simulink subsystem "DesalHydraulicsERU"  (R2025b)
settings: Solver=VariableStepAuto  StartTime=0.0  StopTime=10.0  RelTol=1e-3
libraries: customization_lib x22, nesl_utility x10, fl_lib x1
settings Model: Creator=ndegoede  LastModifiedBy=degoede

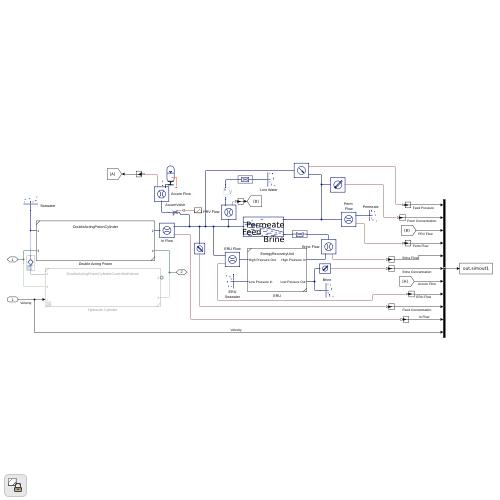
[thumbnail: Simulink's stored preview of the top-level diagram]
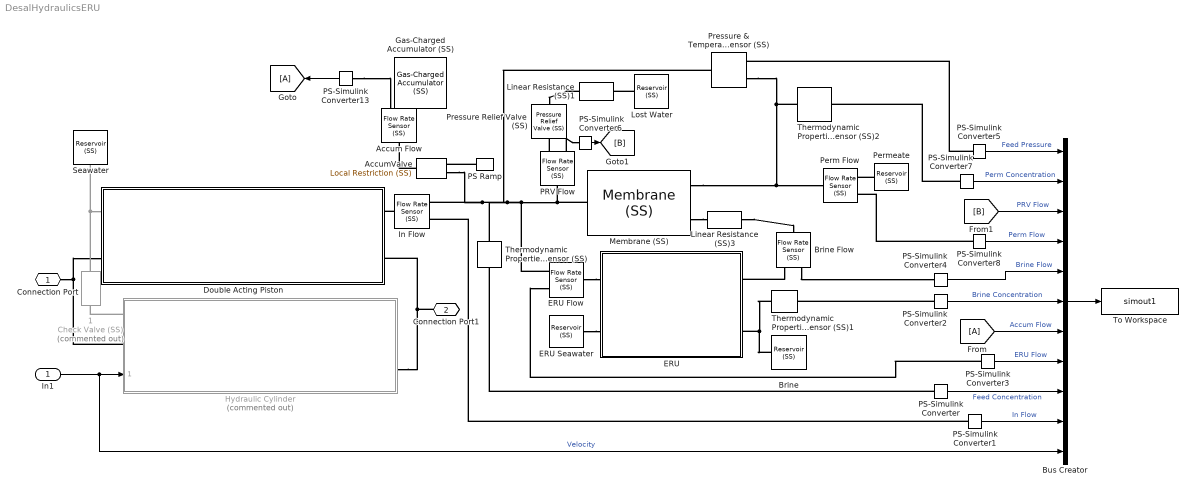
== system DesalHydraulicsERU ==
  In1 : Inport
  " Seawater" : customization_lib/solution/elements/Reservoir (SS)  pressure_spec=foundation.enum.pressure_spec.specified  reservoir_pressure=0.2 MPa  reservoir_temperature=293.15 K  reservoir_concentration=36 kg/m^3  reservoir_concentration_y=0 kg/m^3  reservoir_concentration_z=0 kg/m^3  area=0.01 m^2  custom_ports=false  length_A=1e-3 m
      settings: SourceProductName=Customization  InternalSimscapePortConfiguration="{\"Bottom\":[],\"Left\":[{\"id\":\"A\",\"label\":\"A\",\"type\":\"customization.solution.solution\"}],\"Right\":[],\"Top\":[]}"
  " 1" : customization_lib/solution/elements/Check Valve (SS)  Commented=on  opening_spec=fluids.thermal_liquid.valves.enum.PressureOpeningSpec.Linear  pressure_spec=fluids.thermal_liquid.valves.enum.PressureControlSpec.PressureDifferential  p_crack_gauge=0.1 MPa  p_crack_differential=0.01 MPa  press_max_gauge=0.2 MPa  press_max_differential=0.02 MPa  area_max=0.05 m^2  area_leak=1e-8 m^2  p_diff_TLU=[0.01 : 0.01 : 0.1] MPa  valve_area_TLU=[1e-10, 1e-05, 2e-05, 3e-05, 4e-05, 5e-05, 6e-05, 7.5e-05, 8.5e-05, .0001] m^2  vol_flow_TLU=[.000358, .045, .11, .191, .284, .39, .505, .63, .764, .905] .* 1e-3 m^3/s  area=0.1 m^2  Cd=0.7  Re_c=150  smoothing_factor=0.01  pressure_recovery=false  opening_dynamics=false  tau=0.1 s  custom_ports=false  length_A=1e-3 m  length_B=1e-3 m
      settings: SourceProductName=Customization  InternalSimscapePortConfiguration="{\"Bottom\":[],\"Left\":[{\"id\":\"A\",\"label\":\"A\",\"type\":\"customization.solution.solution\"}],\"Right\":[{\"id\":\"B\",\"label\":\"B\",\"type\":\"customization.solution.solution\"}],\"Top\":[]}"
  Accum Flow : customization_lib/solution/sensors/Flow Rate Sensor (SS)  mass_flow_measure=false  volumetric_flow_measure=true  solute_flow_measure=false  solute_y_flow_measure=false  solute_z_flow_measure=false  energy_flow_measure=false
      settings: SourceProductName=Customization  InternalSimscapePortConfiguration="{\"Bottom\":[],\"Left\":[{\"id\":\"A\",\"label\":\"A\",\"type\":\"customization.solution.solution\"}],\"Right\":[{\"id\":\"B\",\"label\":\"B\",\"type\":\"customization.solution.solution\"},{\"id\":\"V\",\"label\":\"V\",\"type\":\"output\"}],\"Top\":[]}"
  AccumValve : customization_lib/solution/elements/Local Restriction (SS)  restriction_type=foundation.enum.restriction_type.variable  restriction_area=0.001 m^2  min_area=1e-8 m^2  max_area=0.05 m^2  area=0.1 m^2  Cd=0.7  Re_c=150  pressure_recovery=simscape.enum.onoff.off  custom_ports=false  length_A=1e-3 m  length_B=1e-3 m
      settings: SourceProductName=Customization  InternalSimscapePortConfiguration="{\"Bottom\":[],\"Left\":[{\"id\":\"A\",\"label\":\"A\",\"type\":\"customization.solution.solution\"},{\"id\":\"area_in\",\"label\":\"AR\",\"type\":\"input\"}],\"Right\":[{\"id\":\"B\",\"label\":\"B\",\"type\":\"customization.solution.solution\"}],\"Top\":[]}"
  Brine : customization_lib/solution/elements/Reservoir (SS)  pressure_spec=foundation.enum.pressure_spec.atmospheric  reservoir_pressure=0.101325 MPa  reservoir_temperature=293.15 K  reservoir_concentration=36 kg/m^3  reservoir_concentration_y=0 kg/m^3  reservoir_concentration_z=0 kg/m^3  area=0.1 m^2  custom_ports=true  length_A=1 m
      settings: SourceProductName=Customization  InternalSimscapePortConfiguration="{\"Bottom\":[],\"Left\":[{\"id\":\"A\",\"label\":\"A\",\"type\":\"customization.solution.solution\"}],\"Right\":[],\"Top\":[]}"
  Brine Flow : customization_lib/solution/sensors/Flow Rate Sensor (SS)  mass_flow_measure=false  volumetric_flow_measure=true  solute_flow_measure=false  solute_y_flow_measure=false  solute_z_flow_measure=false  energy_flow_measure=false
      settings: SourceProductName=Customization  InternalSimscapePortConfiguration="{\"Bottom\":[],\"Left\":[{\"id\":\"A\",\"label\":\"A\",\"type\":\"customization.solution.solution\"}],\"Right\":[{\"id\":\"B\",\"label\":\"B\",\"type\":\"customization.solution.solution\"},{\"id\":\"V\",\"label\":\"V\",\"type\":\"output\"}],\"Top\":[]}"
  Bus Creator : BusCreator  Inputs=11
  Double Acting Piston : Subsystem  ReferencedSubsystem=DoubleActingPistonCylinder
      settings: PortSchema="{\"entries\":[{\"content\":{\"sides\":[{\"content\":{\"connectorIds\":[\"LConn1\",\"LConn3\"]},\"type\":\"ConnectorPlacement.EquallySpacedRectSide\",\"uuid\":\"8acd0945-963f-4ac9-9e22-6ebef24fa469\"},{\"content\":{\"connectorIds\":[\"LConn2\",\"LConn4\"],\"side\":\"RIGHT\"},\"type\":\"ConnectorPlacement.EquallySpacedRectSide\",\"uuid\":\"3b4a74cd-deb1-4dcf-bacc-c9108daeb4d0\"},{\"content\":{\"side\":\"TOP\"},\"type\":\"ConnectorPlacement.EquallySpacedRectSide\",\"uuid\":\"b26b8698-1eb6-4b70-b966-bc7275cbd4a0\"},{\"content\":{\"side\":\"BOTTOM\"},\"type\":\"ConnectorPlacement.EquallySpacedRectSide\",\"uuid\":\"df97d8fb-7bd4-42c8-81cb-d93f7329400b\"}]},\"type\":\"ConnectorPlacement.EquallySpacedConnector\",\"uuid\":\"8ea66071-78df-4809-a2e0-9adf4b1871fd\"}],\"packageUris\":[\"http://schema.mathworks.com/mf0/Connector/R2020b\"],\"version\":\"1.0\"}"
  ERU : Subsystem  ReferencedSubsystem=EnergyRecoveryUnit
      settings: PortSchema="{\"entries\":[{\"content\":{\"sides\":[{\"content\":{\"connectorIds\":[\"LConn4\",\"LConn3\"]},\"type\":\"ConnectorPlacement.EquallySpacedRectSide\",\"uuid\":\"dfa76b21-2359-4361-afcd-412f59dbf2f7\"},{\"content\":{\"connectorIds\":[\"LConn1\",\"LConn2\"],\"side\":\"RIGHT\"},\"type\":\"ConnectorPlacement.EquallySpacedRectSide\",\"uuid\":\"8a873e0a-23e4-4021-8054-e473ffd3fddb\"},{\"content\":{\"side\":\"TOP\"},\"type\":\"ConnectorPlacement.EquallySpacedRectSide\",\"uuid\":\"dbbe8b32-d4e5-4ced-b70e-6884432bc55a\"}]},\"type\":\"ConnectorPlacement.EquallySpacedConnector\",\"uuid\":\"6b5e7d52-c55b-4be9-b32d-a2c1e9796720\"}],\"packageUris\":[\"http://schema.mathworks.com/mf0/Connector/R2020b\"],\"version\":\"1.0\"}"
  ERU Seawater : customization_lib/solution/elements/Reservoir (SS)  pressure_spec=foundation.enum.pressure_spec.atmospheric  reservoir_pressure=1 MPa  reservoir_temperature=293.15 K  reservoir_concentration=36 kg/m^3  reservoir_concentration_y=0 kg/m^3  reservoir_concentration_z=0 kg/m^3  area=0.1 m^2  custom_ports=true  length_A=1 m
      settings: SourceProductName=Customization  InternalSimscapePortConfiguration="{\"Bottom\":[],\"Left\":[{\"id\":\"A\",\"label\":\"A\",\"type\":\"customization.solution.solution\"}],\"Right\":[],\"Top\":[]}"
  ERU Flow : customization_lib/solution/sensors/Flow Rate Sensor (SS)  mass_flow_measure=false  volumetric_flow_measure=true  solute_flow_measure=false  solute_y_flow_measure=false  solute_z_flow_measure=false  energy_flow_measure=false
      settings: SourceProductName=Customization  InternalSimscapePortConfiguration="{\"Bottom\":[],\"Left\":[{\"id\":\"A\",\"label\":\"A\",\"type\":\"customization.solution.solution\"}],\"Right\":[{\"id\":\"B\",\"label\":\"B\",\"type\":\"customization.solution.solution\"},{\"id\":\"V\",\"label\":\"V\",\"type\":\"output\"}],\"Top\":[]}"
  From : From
  Gas-Charged Accumulator (SS) : customization_lib/solution/elements/Gas-Charged Accumulator (SS)  capacity=4 m^3  dead_volume=4e-5 m^3  p_precharge_gauge=3 MPa  k_sh=1.4  area=0.1 m^2  stiff_coeff=1e7 MPa/m^3  damping_coeff=1e7 MPa*s/m^6  custom_ports=true  length_A=1 m  liquid_volume_specify=off  liquid_volume_priority=High  liquid_volume=5e-3 m^3  liquid_volume_nominal_specify=off  liquid_volume_nominal_value=1  liquid_volume_nominal_unit=m^3  liquid_mass_specify=off  liquid_mass_priority=None  liquid_mass=5 kg  liquid_mass_nominal_specify=off  liquid_mass_nominal_value=1  liquid_mass_nominal_unit=kg  p_I_specify=off  p_I_priority=High  p_I=4 MPa  p_I_nominal_specify=off  p_I_nominal_value=1  p_I_nominal_unit=MPa  T_I_specify=off  T_I_priority=High  T_I=293.15 K  T_I_nominal_specify=off  T_I_nominal_value=1  T_I_nominal_unit=K  x_I_specify=on  x_I_priority=High  x_I=36 kg/m^3  x_I_nominal_specify=off  x_I_nominal_value=1  x_I_nominal_unit=kg/m^3  y_I_specify=off  y_I_priority=High  y_I=0 kg/m^3  y_I_nominal_specify=off  y_I_nominal_value=1  y_I_nominal_unit=kg/m^3  z_I_specify=off  z_I_priority=High  z_I=0 kg/m^3  z_I_nominal_specify=off  z_I_nominal_value=1  z_I_nominal_unit=kg/m^3
      settings: SourceProductName=Customization  InternalSimscapePortConfiguration="{\"Bottom\":[],\"Left\":[],\"Right\":[{\"id\":\"A\",\"label\":\"A\",\"type\":\"customization.solution.solution\"},{\"id\":\"H\",\"label\":\"H\",\"type\":\"foundation.thermal.thermal\"}],\"Top\":[]}"
  Goto : Goto
  Hydraulic Cylinder : Subsystem  Commented=on  ReferencedSubsystem=DoubleActingPistonCylinderControlledValves
      settings: PortSchema="{\"entries\":[{\"content\":{\"sides\":[{\"content\":{\"connectorIds\":[\"LConn1\",\"LConn3\",\"In1\"]},\"type\":\"ConnectorPlacement.EquallySpacedRectSide\",\"uuid\":\"aba0d450-13fa-47c5-97c7-b10a0315f51f\"},{\"content\":{\"connectorIds\":[\"LConn2\",\"LConn4\"],\"side\":\"RIGHT\"},\"type\":\"ConnectorPlacement.EquallySpacedRectSide\",\"uuid\":\"108d113a-e289-4033-b499-0480e5177dd7\"},{\"content\":{\"side\":\"TOP\"},\"type\":\"ConnectorPlacement.EquallySpacedRectSide\",\"uuid\":\"f504290e-6e3f-472e-a0d8-1d71d9a13575\"}]},\"type\":\"ConnectorPlacement.EquallySpacedConnector\",\"uuid\":\"d4991c48-9204-476d-9d46-88f1a2d0e489\"}],\"packageUris\":[\"http://schema.mathworks.com/mf0/Connector/R2020b\"],\"version\":\"1.0\"}"
  In Flow : customization_lib/solution/sensors/Flow Rate Sensor (SS)  mass_flow_measure=false  volumetric_flow_measure=true  solute_flow_measure=false  solute_y_flow_measure=false  solute_z_flow_measure=false  energy_flow_measure=false
      settings: SourceProductName=Customization  InternalSimscapePortConfiguration="{\"Bottom\":[],\"Left\":[{\"id\":\"A\",\"label\":\"A\",\"type\":\"customization.solution.solution\"}],\"Right\":[{\"id\":\"B\",\"label\":\"B\",\"type\":\"customization.solution.solution\"},{\"id\":\"V\",\"label\":\"V\",\"type\":\"output\"}],\"Top\":[]}"
  Linear Resistance (SS)1 : customization_lib/solution/elements/Linear Resistance (SS)  R=60e2 Pa*s/m^3  area=0.1 m^2  custom_ports=true  length_A=1 m  length_B=1 m
      settings: SourceProductName=Customization  InternalSimscapePortConfiguration="{\"Bottom\":[],\"Left\":[{\"id\":\"A\",\"label\":\"A\",\"type\":\"customization.solution.solution\"}],\"Right\":[{\"id\":\"B\",\"label\":\"B\",\"type\":\"customization.solution.solution\"}],\"Top\":[]}"
  Linear Resistance (SS)3 : customization_lib/solution/elements/Linear Resistance (SS)  R=60.23/22 MPa*s/m^3  area=0.1 m^2  custom_ports=true  length_A=1 m  length_B=1 m
      settings: SourceProductName=Customization  InternalSimscapePortConfiguration="{\"Bottom\":[],\"Left\":[{\"id\":\"A\",\"label\":\"A\",\"type\":\"customization.solution.solution\"}],\"Right\":[{\"id\":\"B\",\"label\":\"B\",\"type\":\"customization.solution.solution\"}],\"Top\":[]}"
  Lost Water : customization_lib/solution/elements/Reservoir (SS)  pressure_spec=foundation.enum.pressure_spec.atmospheric  reservoir_pressure=0.101325 MPa  reservoir_temperature=293.15 K  reservoir_concentration=36 kg/m^3  reservoir_concentration_y=0 kg/m^3  reservoir_concentration_z=0 kg/m^3  area=0.1 m^2  custom_ports=true  length_A=1 m
      settings: SourceProductName=Customization  InternalSimscapePortConfiguration="{\"Bottom\":[],\"Left\":[{\"id\":\"A\",\"label\":\"A\",\"type\":\"customization.solution.solution\"}],\"Right\":[],\"Top\":[]}"
  Membrane (SS) : customization_lib/membranes/Membrane (SS)  A_w=2.57e-12 m^3/(N*s)  B_s=2.30e-8 m/s  B_s_y=2.30e-8 m/s  B_s_z=2.30e-8 m/s  A_table=[2.57e-12, 2.57e-12, 2.57e-12] m^3/(N*s)  B_table=[2.3e-08, 2.3e-08, 2.3e-08] m/s  B_table_y=[2.3e-08, 2.3e-08, 2.3e-08] m/s  B_table_z=[2.3e-08, 2.3e-08, 2.3e-08] m/s  NDP_index=[.1, 2, 5] MPa  A_m=35.3*183 m^2  length=1 m  D_feed=0.7556 mm  area_feed=21158*183 mm^2  D_perm=29*183^0.376 mm  N=10  coefficient_type=foundation.enum.constant_variable.constant  polarization_type=customization.membranes.polarization_options.none  boundary_height=1 mm  Re_min=0.1  dynamic_compressibility=true  P0_feed=0.101325 MPa  P0_perm=0.101325 MPa  x0_feed=0.2 kg/m^3  x0_perm=0.2 kg/m^3  y0_feed=0 kg/m^3  y0_perm=0 kg/m^3  z0_feed=0 kg/m^3  z0_perm=0 kg/m^3  custom_ports=true  length_A_feed=1 m  length_B_feed=1 m  length_A_perm=1 m  length_B_perm=1 m  boundary_port_length=1 mm  scaling_x=false  x_eq=1e15 g/l  K_G_x=0 m/s  s_x=1  A_nucleation_x=1e-30 m^2  aspect_ratio_x=0.9  scales_per_area_x=0 1/cm^2  alpha_x=1000 1/m  F_detach_x=1 Pa  F_detach_buffer_x=1e-3 N  Mscale_x0=0 kg  scaling_y=false  y_eq=1e15 g/l  K_G_y=0 m/s  s_y=1  A_nucleation_y=1e-30 m^2  aspect_ratio_y=0.9  scales_per_area_y=0 1/cm^2  alpha_y=1000 1/m  F_detach_y=1 Pa  F_detach_buffer_y=1e-3 N  Mscale_y0=0 kg  scaling_z=false  z_eq=1e15 g/l  K_G_z=0 m/s  s_z=1  A_nucleation_z=1e-30 m^2  aspect_ratio_z=0.9  scales_per_area_z=0 1/cm^2  alpha_z=1000 1/m  F_detach_z=1 Pa  F_detach_buffer_z=1e-3 N  Mscale_z0=0 kg
      settings: SourceProductName=Customization  InternalSimscapePortConfiguration="{\"Bottom\":[],\"Left\":[{\"id\":\"F\",\"label\":\"Feed\",\"type\":\"customization.solution.solution\"}],\"Right\":[{\"id\":\"B\",\"label\":\"Brine\",\"type\":\"customization.solution.solution\"},{\"id\":\"P\",\"label\":\"Permeate\",\"type\":\"customization.solution.solution\"}],\"Top\":[]}"
  PRV Flow : customization_lib/solution/sensors/Flow Rate Sensor (SS)  mass_flow_measure=false  volumetric_flow_measure=true  solute_flow_measure=false  solute_y_flow_measure=false  solute_z_flow_measure=false  energy_flow_measure=false
      settings: SourceProductName=Customization  InternalSimscapePortConfiguration="{\"Bottom\":[],\"Left\":[{\"id\":\"A\",\"label\":\"A\",\"type\":\"customization.solution.solution\"}],\"Right\":[{\"id\":\"B\",\"label\":\"B\",\"type\":\"customization.solution.solution\"},{\"id\":\"V\",\"label\":\"V\",\"type\":\"output\"}],\"Top\":[]}"
  PS Ramp : fl_lib/Physical Signals/Sources/PS Ramp  slope=0.05/20 m^2/s  start_time=60 s  initial_output=0  ZeroCross=true
  PS-Simulink Converter{,1..8,13} (10 alike) : nesl_utility/PS-Simulink Converter  PhysicalDomain=network_engine_domain  SubClassName=ps_output  LeftPortType=input  RightPortType=output  PseudoPeriodic=off  Frequencies=[]  VectorFormat=inherit  Unit=inherit  AffineConversion=off
  Perm Flow : customization_lib/solution/sensors/Flow Rate Sensor (SS)  mass_flow_measure=false  volumetric_flow_measure=true  solute_flow_measure=false  solute_y_flow_measure=false  solute_z_flow_measure=false  energy_flow_measure=false
      settings: SourceProductName=Customization  InternalSimscapePortConfiguration="{\"Bottom\":[],\"Left\":[{\"id\":\"A\",\"label\":\"A\",\"type\":\"customization.solution.solution\"}],\"Right\":[{\"id\":\"B\",\"label\":\"B\",\"type\":\"customization.solution.solution\"},{\"id\":\"V\",\"label\":\"V\",\"type\":\"output\"}],\"Top\":[]}"
  Permeate : customization_lib/solution/elements/Reservoir (SS)  pressure_spec=foundation.enum.pressure_spec.specified  reservoir_pressure=0.101325 MPa  reservoir_temperature=293.15 K  reservoir_concentration=0.2 kg/m^3  reservoir_concentration_y=0 kg/m^3  reservoir_concentration_z=0 kg/m^3  area=0.1 m^2  custom_ports=true  length_A=1 m
      settings: SourceProductName=Customization  InternalSimscapePortConfiguration="{\"Bottom\":[],\"Left\":[{\"id\":\"A\",\"label\":\"A\",\"type\":\"customization.solution.solution\"}],\"Right\":[],\"Top\":[]}"
  Pressure & Temperature Sensor (SS) : customization_lib/solution/sensors/Pressure & Temperature Sensor (SS)  reference=foundation.enum.MeasurementReference.difference  pressure=true  pressure_spec=foundation.enum.PressureMeasementSpec.Absolute  temperature=false
      settings: SourceProductName=Customization  InternalSimscapePortConfiguration="{\"Bottom\":[],\"Left\":[{\"id\":\"A\",\"label\":\"A\",\"type\":\"customization.solution.solution\"}],\"Right\":[{\"id\":\"B\",\"label\":\"B\",\"type\":\"customization.solution.solution\"},{\"id\":\"P\",\"label\":\"P\",\"type\":\"output\"}],\"Top\":[]}"
  Pressure Relief Valve (SS) : customization_lib/solution/elements/Pressure Relief Valve (SS)  set_pressure=5.6 MPa  reg_range=0.1 MPa  max_area=2.67e-2 m^2  min_area=1e-6 m^2  area=0.1 m^2  Cd=0.7  Re_c=150  custom_ports=true  delay_time=0.1 s  length_A=1 m  length_B=1 m
      settings: SourceProductName=Customization  InternalSimscapePortConfiguration="{\"Bottom\":[],\"Left\":[{\"id\":\"A\",\"label\":\"A\",\"type\":\"customization.solution.solution\"}],\"Right\":[{\"id\":\"B\",\"label\":\"B\",\"type\":\"customization.solution.solution\"}],\"Top\":[]}"
  Thermodynamic Properties Sensor (SS) : customization_lib/solution/sensors/Thermodynamic Properties Sensor (SS)  density_measure=false  concentration_measure=true  concentration_y_measure=false  concentration_z_measure=false
      settings: SourceProductName=Customization  InternalSimscapePortConfiguration="{\"Bottom\":[],\"Left\":[{\"id\":\"A\",\"label\":\"A\",\"type\":\"customization.solution.solution\"}],\"Right\":[{\"id\":\"X\",\"label\":\"X\",\"type\":\"output\"}],\"Top\":[]}"
  Thermodynamic Properties Sensor (SS)1 : customization_lib/solution/sensors/Thermodynamic Properties Sensor (SS)  density_measure=false  concentration_measure=true  concentration_y_measure=false  concentration_z_measure=false
      settings: SourceProductName=Customization  InternalSimscapePortConfiguration="{\"Bottom\":[],\"Left\":[{\"id\":\"A\",\"label\":\"A\",\"type\":\"customization.solution.solution\"}],\"Right\":[{\"id\":\"X\",\"label\":\"X\",\"type\":\"output\"}],\"Top\":[]}"
  Thermodynamic Properties Sensor (SS)2 : customization_lib/solution/sensors/Thermodynamic Properties Sensor (SS)  density_measure=false  concentration_measure=true  concentration_y_measure=false  concentration_z_measure=false
      settings: SourceProductName=Customization  InternalSimscapePortConfiguration="{\"Bottom\":[],\"Left\":[{\"id\":\"A\",\"label\":\"A\",\"type\":\"customization.solution.solution\"}],\"Right\":[{\"id\":\"X\",\"label\":\"X\",\"type\":\"output\"}],\"Top\":[]}"
  To Workspace : ToWorkspace  VariableName=simout1  SaveFormat=Timeseries  SampleTime=-1
  Connection Port : PMIOPort  Side=Left
  Connection Port1 : PMIOPort  Port=2  Side=Left
  wires:
  Bus Creator/1 -> To Workspace/1
  PS-Simulink Converter2/1 -> Bus Creator/6  "Brine Concentration"
  PS-Simulink Converter7/1 -> Bus Creator/2  "Perm Concentration"
  PS-Simulink Converter5/1 -> Bus Creator/1  "Feed Pressure"
  PS-Simulink Converter/1 -> Bus Creator/9  "Feed Concentration"
  PS-Simulink Converter8/1 -> Bus Creator/4  "Perm Flow"
  PS-Simulink Converter1/1 -> Bus Creator/10  "In Flow"
  PS-Simulink Converter6/1 -> [B]
  PS-Simulink Converter13/1 -> Goto/1
  From/1 -> Bus Creator/7  "Accum Flow"
  PS-Simulink Converter3/1 -> Bus Creator/8  "ERU Flow"
  [B] -> Bus Creator/3  "PRV Flow"
  In1/1 -> Bus Creator/11, Hydraulic Cylinder/1  "Velocity"
  PS-Simulink Converter4/1 -> Bus Creator/5  "Brine Flow"
  connections:
  Thermodynamic Properties Sensor (SS)1/LConn1 -- ERU/LConn2 -- Brine/LConn1
  Connection Port1/RConn1 -- Hydraulic Cylinder/LConn4 -- Double Acting Piston/LConn4
  Connection Port/RConn1 -- Hydraulic Cylinder/LConn3 -- Double Acting Piston/LConn3
  Pressure & Temperature Sensor (SS)/RConn1 -- Membrane (SS)/RConn2 -- Perm Flow/LConn1 -- Thermodynamic Properties Sensor (SS)2/LConn1
  Membrane (SS)/LConn1 -- Thermodynamic Properties Sensor (SS)/LConn1 -- In Flow/RConn1 -- AccumValve/LConn1 -- Pressure & Temperature Sensor (SS)/LConn1 -- ERU Flow/RConn1 -- PRV Flow/LConn1
  " 1"/LConn1 -- " Seawater"/LConn1 -- Double Acting Piston/LConn1
  ERU Seawater/LConn1 -- ERU/LConn3
  Permeate/LConn1 -- Perm Flow/RConn1
  Brine Flow/RConn1 -- ERU/LConn1
  PRV Flow/RConn1 -- Pressure Relief Valve (SS)/LConn1
  Linear Resistance (SS)1/LConn1 -- Pressure Relief Valve (SS)/RConn1
  Lost Water/LConn1 -- Linear Resistance (SS)1/RConn1
  PS-Simulink Converter2/LConn1 -- Thermodynamic Properties Sensor (SS)1/RConn1
  PS-Simulink Converter5/LConn1 -- Pressure & Temperature Sensor (SS)/RConn2
  PRV Flow/RConn2 -- PS-Simulink Converter6/LConn1
  PS-Simulink Converter7/LConn1 -- Thermodynamic Properties Sensor (SS)2/RConn1
  PS-Simulink Converter8/LConn1 -- Perm Flow/RConn2
  PS-Simulink Converter13/LConn1 -- Accum Flow/RConn2
  ERU Flow/LConn1 -- ERU/LConn4
  PS-Simulink Converter3/LConn1 -- ERU Flow/RConn2
  PS-Simulink Converter1/LConn1 -- In Flow/RConn2
  PS-Simulink Converter/LConn1 -- Thermodynamic Properties Sensor (SS)/RConn1
  Accum Flow/RConn1 -- Gas-Charged Accumulator (SS)/RConn1
  Linear Resistance (SS)3/RConn1 -- Brine Flow/LConn1
  Membrane (SS)/RConn1 -- Linear Resistance (SS)3/LConn1
  Hydraulic Cylinder/LConn1 -- " 1"/RConn1
  In Flow/LConn1 -- Double Acting Piston/LConn2
  Brine Flow/RConn2 -- PS-Simulink Converter4/LConn1
  PS Ramp/RConn1 -- AccumValve/LConn2
  AccumValve/RConn1 -- Accum Flow/LConn1
